simulink model "tqdtqr_rebuild_V3"  (R2021b)
settings: Solver=VariableStepAuto  StartTime=0.0  StopTime=10.0  RelTol=1e-3
undefined symbols (not defined in the file): ATQD_AfterTqMinGain_X_Deg, ATQD_APSCreepBaseTqD_X_kph, ATQD_APSCreepBaseTqD_Y_Deg, ATQD_APSCreepBaseTqR_X_kph, ATQD_APSCreepBaseTqR_Y_Deg, ATQD_APSCreepIterm_X_kph, ATQD_APSCreepIterm_Y_kph, ATQD_APSCreepPterm_X_kph, ATQD_APSCreepPterm_Y_kph, ATQD_APSDecReq_X_kph, ATQD_APSDecReq_Y_mps2, ATQD_APSDecReqCMD_X_kph, ATQD_APSDecReqTs_X_pct, ATQD_APSDecTimeGain_X_Deg, ATQD_APSDecTimeGain_Y_s, ATQD_APSReqLowSpd_X_Deg, ATQD_AutoHoldReleaseBPS_X_Deg, ATQD_AWDLoadTrqnsGain_X_kg, ATQD_AWDLoadTrqnsGain_Y_pct, ATQD_BOSEnBPSPosn_X_kph, ATQD_BOSMap_X_rpm, ATQD_BOSMap_Y_pct, ATQD_CreepBaseTqD_X_kph, ATQD_CreepBaseTqD_Y_Deg, ATQD_CreepBaseTqR_X_kph, ATQD_CreepBaseTqR_Y_Deg, ATQD_CreepBPSDisPosn_X_Deg, ATQD_CreepBPSDisPosnR_X_Deg, ATQD_CreepBPSEnPosn_X_Deg, ATQD_CreepBPSEnPosnR_X_Deg, ATQD_CreepDeltaTq_X_kph, ATQD_CreepIterm_X_kph, ATQD_CreepIterm_Y_kph, ATQD_CreepItermMaxLimit_X_pct, ATQD_CreepPreloadTime_X_kph, ATQD_CreepPreloadTq_X_kph, ATQD_CreepPreloadTq_Y_s, ATQD_CreepProtTq_X_Deg, ATQD_CreepPterm_X_kph, ATQD_CreepPterm_Y_kph, ATQD_CreepRrTqSpRat_X_rpm, ATQD_CreepRrTqSpRat_Y_Nm, ATQD_CreepTargetSpdD_X_pct, ATQD_CreepTargetSpdR_X_pct, ATQD_CreepUpLimitTq_X_rpm, ATQD_DecIneOPDHoldEnDelay_X_Deg, ATQD_DecIneOPDHoldEnDelay_Y_bar, ATQD_ECOTqMapD_X_rpm, ATQD_ECOTqMapD_Y_pct, ATQD_EMTqMapD_X_rpm, ATQD_EMTqMapD_Y_pct, ATQD_EOPDTqMapDCon_X_rpm, ATQD_EOPDTqMapDCon_Y_Deg, ATQD_EstInitVehWeight_X_c, ATQD_FAfterTqCMDGain_X_rpm, ATQD_FAfterTqCMDGain_Y_pct, ATQD_ForceLowSpd_X_Deg, ATQD_ForcePLimitSpd_X_Deg, ATQD_FrLossMAPLowV_X_rpm, ATQD_FrLossMAPLowV_Y_Nm ... (+949)
libraries: simulink x235, hcu_lib x208, tqr x63, tqd x6
(part 27 of 37)

== system tqdtqr_rebuild_V3/Input_Convert/Main function/Front//Rear ramp parameters determine/Front wheel rate limit determination/VTQR_VMCFEDUIncDec_Nm ==
  VTQR_FEDUWhlTqReqSmoothDelay_Nm : Inport
  VTQD_TqTargetShaftSpd_rpm : Inport  Port=2
  Action Port : ActionPort  ActionPortLabel=elseif(u4~=0)
  Data Type Conversion1 : DataTypeConversion  OutDataTypeStr=single
  Data Type Conversion2 : DataTypeConversion  OutDataTypeStr=single
  Data Type Conversion3 : DataTypeConversion  OutDataTypeStr=single
  MTQR_VMCFEDUTqDecSR_Z_Nm1 : Lookup_n-D  BreakpointsForDimension1=ATQR_VMCFEDUTqIncSR_Y_Nm  BreakpointsForDimension2=ATQR_VMCFEDUTqIncSR_X_rpm  Table=MTQR_VMCFEDUTqDecSR_Z_Nm  ExtrapMethod=Clip  InternalRulePriority=Speed  RndMeth=Simplest  InputSameDT=on
      settings: InputPortMap=u0,u1
  MTQR_VMCFEDUTqIncSR_Z_Nm1 : Lookup_n-D  BreakpointsForDimension1=ATQR_VMCFEDUTqIncSR_Y_Nm  BreakpointsForDimension2=ATQR_VMCFEDUTqIncSR_X_rpm  Table=MTQR_VMCFEDUTqIncSR_Z_Nm  ExtrapMethod=Clip  InternalRulePriority=Speed  RndMeth=Simplest  InputSameDT=on
      settings: InputPortMap=u0,u1
  Mux : Mux  Inputs=2
  VTQR_VMCFEDUIncDec_Nm : Outport
  VTQR_VMCFEDUIncDec_Nm1 : Outport  Port=2
  wires:
  [VTQD_TqTargetShaftSpd_rpm] -> MTQR_VMCFEDUTqDecSR_Z_Nm1/2
  [VTQR_FEDUWhlTqReqSmoothDelay_Nm] -> MTQR_VMCFEDUTqDecSR_Z_Nm1/1
  [VTQD_TqTargetShaftSpd_rpm] -> MTQR_VMCFEDUTqIncSR_Z_Nm1/2
  [VTQR_FEDUWhlTqReqSmoothDelay_Nm] -> MTQR_VMCFEDUTqIncSR_Z_Nm1/1
  VTQR_FEDUWhlTqReqSmoothDelay_Nm/1 -> [VTQR_FEDUWhlTqReqSmoothDelay_Nm]
  VTQD_TqTargetShaftSpd_rpm/1 -> [VTQD_TqTargetShaftSpd_rpm]
  [VTQR_VMCFEDUTqIncSR_Nm] -> Data Type Conversion1/1
  [VTQR_VMCFEDUTqDecSR_Nm] -> Data Type Conversion2/1
  Mux/1 -> VTQR_VMCFEDUIncDec_Nm/1
  MTQR_VMCFEDUTqIncSR_Z_Nm1/1 -> [VTQR_VMCFEDUTqIncSR_Nm]  "VTQR_VMCFEDUTqIncSR_Nm"
  MTQR_VMCFEDUTqDecSR_Z_Nm1/1 -> [VTQR_VMCFEDUTqDecSR_Nm]  "VTQR_VMCFEDUTqDecSR_Nm"
  Data Type Conversion2/1 -> Mux/2
  Data Type Conversion1/1 -> Mux/1
  Data Type Conversion3/1 -> VTQR_VMCFEDUIncDec_Nm1/1
  [VTQR_VMCFEDUTqDecSR_Nm] -> Data Type Conversion3/1

== system tqdtqr_rebuild_V3/Input_Convert/Main function/Front//Rear ramp parameters determine/Rear First order filter input tau map and determination/VTQR_CreepREDUTs_c ==
  VTQR_REDUWhlTqReqSmooth_Nm : Inport
  VTQD_TqTargetShaftSpd_rpm : Inport  Port=2
  VVMC_EstSlope_Deg : Inport  Port=3
  Action Port : ActionPort  ActionPortLabel=elseif(u2 ~= 0)
  Data Type Conversion : DataTypeConversion  OutDataTypeStr=single
  Data Type Conversion1 : DataTypeConversion  OutDataTypeStr=single
  MTQR_CreepGradeREDUTs_Z_c : Lookup_n-D  BreakpointsForDimension1=ATQR_CreepGradeREDUTs_Y_Deg  BreakpointsForDimension2=ATQR_CreepGradeREDUTs_X_rpm  Table=MTQR_CreepGradeREDUTs_Z_c  ExtrapMethod=Clip  InternalRulePriority=Speed  RndMeth=Simplest  InputSameDT=on
      settings: InputPortMap=u0,u1
  MTQR_CreepREDUTs_Z_c1 : Lookup_n-D  BreakpointsForDimension1=ATQR_CreepFEDUTs_Y_Nm  BreakpointsForDimension2=ATQR_CreepFEDUTs_X_rpm  Table=MTQR_CreepREDUTs_Z_c  ExtrapMethod=Clip  InternalRulePriority=Speed  RndMeth=Simplest  InputSameDT=on
      settings: InputPortMap=u0,u1
  Min : MinMax  Inputs=2
  VTQR_CreepREDUTs_c : Outport
  wires:
  [VTQR_CreepREDUTs_c] -> Data Type Conversion/1
  MTQR_CreepREDUTs_Z_c1/1 -> [VTQR_CreepREDUTs_c]  "VTQR_CreepREDUTs_c"
  VTQR_REDUWhlTqReqSmooth_Nm/1 -> [VTQR_REDUWhlTqReqSmooth_Nm]
  VTQD_TqTargetShaftSpd_rpm/1 -> [VTQD_TqTargetShaftSpd_rpm]
  VVMC_EstSlope_Deg/1 -> [VVMC_EstSlope_Deg]
  [VTQD_TqTargetShaftSpd_rpm] -> MTQR_CreepREDUTs_Z_c1/2
  [VTQR_REDUWhlTqReqSmooth_Nm] -> MTQR_CreepREDUTs_Z_c1/1
  [VTQD_TqTargetShaftSpd_rpm] -> MTQR_CreepGradeREDUTs_Z_c/2
  MTQR_CreepGradeREDUTs_Z_c/1 -> [VTQR_CreepGradeREDUTs_c]  "VTQR_CreepGradeREDUTs_c"
  [VVMC_EstSlope_Deg] -> MTQR_CreepGradeREDUTs_Z_c/1
  [VTQR_CreepGradeREDUTs_c] -> Data Type Conversion1/1
  Data Type Conversion/1 -> Min/1
  Data Type Conversion1/1 -> Min/2
  Min/1 -> VTQR_CreepREDUTs_c/1

== system tqdtqr_rebuild_V3/Input_Convert/Main function/Front//Rear ramp parameters determine/Rear First order filter input tau map and determination/VTQR_PreLoadPreEnTs_c ==
  KTQR_PreLoadPreEnTs_c : Inport
  Action Port : ActionPort  ActionPortLabel=elseif(u6~=0)
  VTQR_PreLoadPreEnTs_c : Outport
  wires:
  KTQR_PreLoadPreEnTs_c/1 -> VTQR_PreLoadPreEnTs_c/1

== system tqdtqr_rebuild_V3/Input_Convert/Main function/Front//Rear ramp parameters determine/Rear First order filter input tau map and determination/VTQR_PreLoadTs_c ==
  KTQR_PreLoadTs_c : Inport
  Action Port : ActionPort  ActionPortLabel=elseif(u5~=0)
  VTQR_PreLoadTs_c : Outport
  wires:
  KTQR_PreLoadTs_c/1 -> VTQR_PreLoadTs_c/1

== system tqdtqr_rebuild_V3/Input_Convert/Main function/Front//Rear ramp parameters determine/Rear First order filter input tau map and determination/VTQR_RDCActiveREDUTs_c ==
  VTQD_RegenMode_enum : Inport
  VVMC_ActMaxSlideRate_pct : Inport  Port=2
  Action Port : ActionPort  ActionPortLabel=if(u1~= 0)
  Data Type Conversion : DataTypeConversion  OutDataTypeStr=single
  Data Type Conversion1 : DataTypeConversion  OutDataTypeStr=single
  MTQR_AltRDCActiveREDUTs_Z_c1 : Lookup_n-D  BreakpointsForDimension1=ATQR_AltRDCActiveREDUTs_Y_enum  BreakpointsForDimension2=ATQR_AltRDCActiveREDUTs_X_pct  Table=MTQR_AltRDCActiveREDUTs_Z_c  TableDataTypeStr=Inherit: Inherit from 'Table data'  ExtrapMethod=Clip  InternalRulePriority=Speed  RndMeth=Simplest  InputSameDT=on
      settings: InputPortMap=u0,u1
  VTQR_RDCActiveREDUTs_c : Outport
  wires:
  MTQR_AltRDCActiveREDUTs_Z_c1/1 -> [VTQR_RDCActiveREDUTs_c]  "VTQR_RDCActiveREDUTs_c"
  Data Type Conversion1/1 -> MTQR_AltRDCActiveREDUTs_Z_c1/1
  VTQD_RegenMode_enum/1 -> Data Type Conversion1/1
  VVMC_ActMaxSlideRate_pct/1 -> MTQR_AltRDCActiveREDUTs_Z_c1/2
  [VTQR_RDCActiveREDUTs_c] -> Data Type Conversion/1
  Data Type Conversion/1 -> VTQR_RDCActiveREDUTs_c/1

== system tqdtqr_rebuild_V3/Input_Convert/Main function/Front//Rear ramp parameters determine/Rear First order filter input tau map and determination/VTQR_REDUTIPOutTs_c ==
  VTQD_TqTargetShaftSpd_rpm : Inport
  Action Port : ActionPort  ActionPortLabel=elseif(u4~=0)
  Data Type Conversion : DataTypeConversion  OutDataTypeStr=single
  MTQR_REDUTIPOutTs_Y_c1 : Lookup_n-D  NumberOfTableDimensions=1  BreakpointsForDimension1=ATQR_FEDUTIPOutTs_X_rpm  Table=MTQR_REDUTIPOutTs_Y_c  ExtrapMethod=Clip  InternalRulePriority=Speed  RndMeth=Simplest  InputSameDT=on
  VTQR_REDUTIPOutTs_c : Outport
  wires:
  MTQR_REDUTIPOutTs_Y_c1/1 -> [VTQR_REDUTIPOutTs_c]  "VTQR_REDUTIPOutTs_c"
  VTQD_TqTargetShaftSpd_rpm/1 -> MTQR_REDUTIPOutTs_Y_c1/1
  [VTQR_REDUTIPOutTs_c] -> Data Type Conversion/1
  Data Type Conversion/1 -> VTQR_REDUTIPOutTs_c/1

== system tqdtqr_rebuild_V3/Input_Convert/Main function/Front//Rear ramp parameters determine/Rear First order filter input tau map and determination/VTQR_REDUTs_c ==
  VTQR_REDUTs_c : Inport
  Action Port : ActionPort  ActionPortLabel=else
  VTQR_OutREDUTs_c : Outport
  wires:
  VTQR_REDUTs_c/1 -> VTQR_OutREDUTs_c/1

== system tqdtqr_rebuild_V3/Input_Convert/Main function/Front//Rear ramp parameters determine/Rear First order filter input tau map and determination/VTQR_VMCREDUTs_c ==
  VTQR_REDUWhlTqReqSmooth_Nm : Inport
  VTQD_TqTargetShaftSpd_rpm : Inport  Port=2
  Action Port : ActionPort  ActionPortLabel=elseif( u3 ~= 0)
  Data Type Conversion : DataTypeConversion  OutDataTypeStr=single
  MTQR_VMCREDUTs_Z_c1 : Lookup_n-D  BreakpointsForDimension1=ATQR_VMCREDUTs_Y_Nm  BreakpointsForDimension2=ATQR_VMCFEDUTs_X_rpm  Table=MTQR_VMCREDUTs_Z_c  ExtrapMethod=Clip  InternalRulePriority=Speed  RndMeth=Simplest  InputSameDT=on
      settings: InputPortMap=u0,u1
  VTQR_VMCREDUTs_c : Outport
  wires:
  [VTQR_VMCREDUTs_c] -> Data Type Conversion/1
  Data Type Conversion/1 -> VTQR_VMCREDUTs_c/1
  MTQR_VMCREDUTs_Z_c1/1 -> [VTQR_VMCREDUTs_c]  "VTQR_VMCREDUTs_c"
  VTQR_REDUWhlTqReqSmooth_Nm/1 -> MTQR_VMCREDUTs_Z_c1/1
  VTQD_TqTargetShaftSpd_rpm/1 -> MTQR_VMCREDUTs_Z_c1/2

== system tqdtqr_rebuild_V3/Input_Convert/Main function/Front//Rear ramp parameters determine/Rear wheel rate limit determination1/Drive mode ==
  VTQR_DriveModeTqIncDec_Nm : Inport
  Action Port : ActionPort  ActionPortLabel=else
  VTQR_OutDriveModeTqIncDec_Nm : Outport
  wires:
  VTQR_DriveModeTqIncDec_Nm/1 -> VTQR_OutDriveModeTqIncDec_Nm/1

== system tqdtqr_rebuild_V3/Input_Convert/Main function/Front//Rear ramp parameters determine/Rear wheel rate limit determination1/VTQD_OutRrZeroPointIncDec_Nm ==
  VTQD_RrZeroPointIncDec_Nm : Inport
  Action Port : ActionPort  ActionPortLabel=if(u1~= 0)
  VTQD_OutRrZeroPointIncDec_Nm : Outport
  wires:
  VTQD_RrZeroPointIncDec_Nm/1 -> VTQD_OutRrZeroPointIncDec_Nm/1

== system tqdtqr_rebuild_V3/Input_Convert/Main function/Front//Rear ramp parameters determine/Rear wheel rate limit determination1/VTQR_CreepREDUTqIncDecSR_Nm ==
  VTQR_REDUWhlTqReqSmoothDelay_Nm : Inport
  VTQD_TqTargetShaftSpd_rpm : Inport  Port=2
  VVMC_EstSlope_Deg : Inport  Port=3
  Action Port : ActionPort  ActionPortLabel=elseif(u2 ~= 0)
  Data Type Conversion : DataTypeConversion  OutDataTypeStr=single
  Data Type Conversion1 : DataTypeConversion  OutDataTypeStr=single
  MTQR_CreepGradeRTqDecSR_Z_c : Lookup_n-D  BreakpointsForDimension1=ATQR_CreepGradeRTqIncSR_Y_Deg  BreakpointsForDimension2=ATQR_CreepGradeRTqIncSR_X_rpm  Table=MTQR_CreepGradeRTqDecSR_Z_c  ExtrapMethod=Clip  InternalRulePriority=Speed  RndMeth=Simplest  InputSameDT=on
      settings: InputPortMap=u0,u1
  MTQR_CreepGradeRTqIncSR_Z_c : Lookup_n-D  BreakpointsForDimension1=ATQR_CreepGradeRTqIncSR_Y_Deg  BreakpointsForDimension2=ATQR_CreepGradeRTqIncSR_X_rpm  Table=MTQR_CreepGradeRTqIncSR_Z_c  ExtrapMethod=Clip  InternalRulePriority=Speed  RndMeth=Simplest  InputSameDT=on
      settings: InputPortMap=u0,u1
  MTQR_CreepREDUTqDecSR_Z_Nm1 : Lookup_n-D  BreakpointsForDimension1=ATQR_CreepFEDUTqIncSR_Y_Nm  BreakpointsForDimension2=ATQR_CreepFEDUTqIncSR_X_rpm  Table=MTQR_CreepREDUTqDecSR_Z_Nm  ExtrapMethod=Clip  InternalRulePriority=Speed  RndMeth=Simplest  InputSameDT=on
      settings: InputPortMap=u0,u1
  MTQR_CreepREDUTqIncSR_Z_Nm1 : Lookup_n-D  BreakpointsForDimension1=ATQR_CreepFEDUTqIncSR_Y_Nm  BreakpointsForDimension2=ATQR_CreepFEDUTqIncSR_X_rpm  Table=MTQR_CreepREDUTqIncSR_Z_Nm  ExtrapMethod=Clip  InternalRulePriority=Speed  RndMeth=Simplest  InputSameDT=on
      settings: InputPortMap=u0,u1
  Mux : Mux  Inputs=2
  Product : Product
  Product1 : Product
  VTQR_CreepREDUTqIncDecSR_Nm : Outport
  wires:
  VTQR_REDUWhlTqReqSmoothDelay_Nm/1 -> [VTQR_REDUWhlTqReqSmoothDelay_Nm]
  VTQD_TqTargetShaftSpd_rpm/1 -> [VTQD_TqTargetShaftSpd_rpm]
  [VTQD_TqTargetShaftSpd_rpm] -> MTQR_CreepREDUTqIncSR_Z_Nm1/2
  [VTQR_REDUWhlTqReqSmoothDelay_Nm] -> MTQR_CreepREDUTqIncSR_Z_Nm1/1
  [VTQR_REDUWhlTqReqSmoothDelay_Nm] -> MTQR_CreepREDUTqDecSR_Z_Nm1/1
  [VTQD_TqTargetShaftSpd_rpm] -> MTQR_CreepREDUTqDecSR_Z_Nm1/2
  [VTQR_CreepREDUTqIncSR_Nm] -> Data Type Conversion/1
  [VTQR_CreepREDUTqDecSR_Nm] -> Data Type Conversion1/1
  Data Type Conversion/1 -> Mux/1
  Data Type Conversion1/1 -> Mux/2
  Mux/1 -> VTQR_CreepREDUTqIncDecSR_Nm/1
  MTQR_CreepREDUTqIncSR_Z_Nm1/1 -> Product1/1
  [VTQR_CreepGradeRTqIncSR_c] -> Product1/2
  Product1/1 -> [VTQR_CreepREDUTqIncSR_Nm]  "VTQR_CreepREDUTqIncSR_Nm"
  [VVMC_EstSlope_Deg] -> MTQR_CreepGradeRTqDecSR_Z_c/1
  [VVMC_EstSlope_Deg] -> MTQR_CreepGradeRTqIncSR_Z_c/1
  [VTQD_TqTargetShaftSpd_rpm] -> MTQR_CreepGradeRTqDecSR_Z_c/2
  MTQR_CreepGradeRTqDecSR_Z_c/1 -> [VTQR_CreepGradeRTqDecSR_c]  "VTQR_CreepGradeRTqDecSR_c"
  MTQR_CreepGradeRTqIncSR_Z_c/1 -> [VTQR_CreepGradeRTqIncSR_c]  "VTQR_CreepGradeRTqIncSR_c"
  [VTQD_TqTargetShaftSpd_rpm] -> MTQR_CreepGradeRTqIncSR_Z_c/2
  Product/1 -> [VTQR_CreepREDUTqDecSR_Nm]  "VTQR_CreepREDUTqDecSR_Nm"
  MTQR_CreepREDUTqDecSR_Z_Nm1/1 -> Product/1
  [VTQR_CreepGradeRTqDecSR_c] -> Product/2
  VVMC_EstSlope_Deg/1 -> [VVMC_EstSlope_Deg]

== system tqdtqr_rebuild_V3/Input_Convert/Main function/Front//Rear ramp parameters determine/Rear wheel rate limit determination1/VTQR_RrPreLoadTqIncDecSR_Nm ==
  VTQR_REDUWhlTqReqSmoothDelay_Nm : Inport
  VTQD_TqTargetShaftSpd_rpm : Inport  Port=2
  Action Port : ActionPort  ActionPortLabel=elseif( u3 ~= 0)
  Data Type Conversion : DataTypeConversion  OutDataTypeStr=single
  Data Type Conversion1 : DataTypeConversion  OutDataTypeStr=single
  MTQR_RrPreLoadTqDecSR_Z_Nm1 : Lookup_n-D  BreakpointsForDimension1=ATQR_RrPreLoadTqIncSR_Y_Nm  BreakpointsForDimension2=ATQR_RrPreLoadTqIncSR_X_rpm  Table=MTQR_RrPreLoadTqDecSR_Z_Nm  ExtrapMethod=Clip  InternalRulePriority=Speed  RndMeth=Simplest  InputSameDT=on
      settings: InputPortMap=u0,u1
  MTQR_RrPreLoadTqIncSR_Z_Nm1 : Lookup_n-D  BreakpointsForDimension1=ATQR_RrPreLoadTqIncSR_Y_Nm  BreakpointsForDimension2=ATQR_RrPreLoadTqIncSR_X_rpm  Table=MTQR_RrPreLoadTqIncSR_Z_Nm  ExtrapMethod=Clip  InternalRulePriority=Speed  RndMeth=Simplest  InputSameDT=on
      settings: InputPortMap=u0,u1
  Mux : Mux  Inputs=2
  VTQR_RrPreLoadTqIncDecSR_Nm : Outport
  wires:
  Mux/1 -> VTQR_RrPreLoadTqIncDecSR_Nm/1
  Data Type Conversion1/1 -> Mux/2
  Data Type Conversion/1 -> Mux/1
  [VTQR_RrPreLoadTqDecSR_Nm] -> Data Type Conversion1/1
  [VTQR_RrPreLoadTqIncSR_Nm] -> Data Type Conversion/1
  VTQD_TqTargetShaftSpd_rpm/1 -> [VTQD_TqTargetShaftSpd_rpm]
  VTQR_REDUWhlTqReqSmoothDelay_Nm/1 -> [VTQR_REDUWhlTqReqSmoothDelay_Nm]
  MTQR_RrPreLoadTqIncSR_Z_Nm1/1 -> [VTQR_RrPreLoadTqIncSR_Nm]  "VTQR_RrPreLoadTqIncSR_Nm"
  MTQR_RrPreLoadTqDecSR_Z_Nm1/1 -> [VTQR_RrPreLoadTqDecSR_Nm]  "VTQR_RrPreLoadTqDecSR_Nm"
  [VTQR_REDUWhlTqReqSmoothDelay_Nm] -> MTQR_RrPreLoadTqIncSR_Z_Nm1/1
  [VTQD_TqTargetShaftSpd_rpm] -> MTQR_RrPreLoadTqIncSR_Z_Nm1/2
  [VTQR_REDUWhlTqReqSmoothDelay_Nm] -> MTQR_RrPreLoadTqDecSR_Z_Nm1/1
  [VTQD_TqTargetShaftSpd_rpm] -> MTQR_RrPreLoadTqDecSR_Z_Nm1/2

== system tqdtqr_rebuild_V3/Input_Convert/Main function/Front//Rear ramp parameters determine/Rear wheel rate limit determination1/VTQR_VMCREDUTqIncDecSR_Nm ==
  VTQR_REDUWhlTqReqSmoothDelay_Nm : Inport
  VTQD_TqTargetShaftSpd_rpm : Inport  Port=2
  Action Port : ActionPort  ActionPortLabel=elseif( u4~=0)
  Data Type Conversion : DataTypeConversion  OutDataTypeStr=single
  Data Type Conversion1 : DataTypeConversion  OutDataTypeStr=single
  MTQR_VMCREDUTqDecSR_Z_Nm1 : Lookup_n-D  BreakpointsForDimension1=ATQR_VMCREDUTqIncSR_Y_Nm  BreakpointsForDimension2=ATQR_VMCFEDUTqIncSR_X_rpm  Table=MTQR_VMCREDUTqDecSR_Z_Nm  ExtrapMethod=Clip  InternalRulePriority=Speed  RndMeth=Simplest  InputSameDT=on
      settings: InputPortMap=u0,u1
  MTQR_VMCREDUTqIncSR_Z_Nm1 : Lookup_n-D  BreakpointsForDimension1=ATQR_VMCREDUTqIncSR_Y_Nm  BreakpointsForDimension2=ATQR_VMCFEDUTqIncSR_X_rpm  Table=MTQR_VMCREDUTqIncSR_Z_Nm  ExtrapMethod=Clip  InternalRulePriority=Speed  RndMeth=Simplest  InputSameDT=on
      settings: InputPortMap=u0,u1
  Mux : Mux  Inputs=2
  VTQR_VMCREDUTqIncDecSR_Nm : Outport
  VTQR_VMCREDUTqDecSR_Nm : Outport  Port=2
  wires:
  [VTQD_TqTargetShaftSpd_rpm] -> MTQR_VMCREDUTqDecSR_Z_Nm1/2
  [VTQR_REDUWhlTqReqSmoothDelay_Nm] -> MTQR_VMCREDUTqDecSR_Z_Nm1/1
  [VTQD_TqTargetShaftSpd_rpm] -> MTQR_VMCREDUTqIncSR_Z_Nm1/2
  [VTQR_REDUWhlTqReqSmoothDelay_Nm] -> MTQR_VMCREDUTqIncSR_Z_Nm1/1
  VTQR_REDUWhlTqReqSmoothDelay_Nm/1 -> [VTQR_REDUWhlTqReqSmoothDelay_Nm]
  VTQD_TqTargetShaftSpd_rpm/1 -> [VTQD_TqTargetShaftSpd_rpm]
  [VTQR_VMCREDUTqIncSR_Nm] -> Data Type Conversion/1
  [VTQR_VMCREDUTqDecSR_Nm] -> Data Type Conversion1/1
  Data Type Conversion/1 -> Mux/1
  Data Type Conversion1/1 -> Mux/2
  Mux/1 -> VTQR_VMCREDUTqIncDecSR_Nm/1
  MTQR_VMCREDUTqDecSR_Z_Nm1/1 -> [VTQR_VMCREDUTqDecSR_Nm]  "VTQR_VMCREDUTqDecSR_Nm"
  MTQR_VMCREDUTqIncSR_Z_Nm1/1 -> [VTQR_VMCREDUTqIncSR_Nm]  "VTQR_VMCREDUTqIncSR_Nm"
  [VTQR_VMCREDUTqDecSR_Nm] -> VTQR_VMCREDUTqDecSR_Nm/1

== system tqdtqr_rebuild_V3/Input_Convert/Main function/Front//Rear zero point transfer/Negative Rate limit Determination/VTQR_FrNegRateLimitDecE_Nm ==
  VTQD_TqTargetShaftSpd_rpm : Inport
  VTQR_FEDUWhlTqReqSmoothDelay_Nm : Inport  Port=2
  Action Port : ActionPort  ActionPortLabel=elseif(u2 ~= 0)
  MTQR_FrNegRateLimitDecE_Z_Nm : Lookup_n-D  BreakpointsForDimension1=ATQR_FrNegRateLimitIncN_Y_Nm  BreakpointsForDimension2=ATQR_FrNegRateLimitIncN_X_rpm  Table=MTQR_FrNegRateLimitDecE_Z_Nm  ExtrapMethod=Clip  UseLastTableValue=on  InternalRulePriority=Speed  RndMeth=Simplest  InputSameDT=on
      settings: InputPortMap=u0,u1
  VTQR_FrNegRateLimitDecE_Nm : Outport
  wires:
  VTQD_TqTargetShaftSpd_rpm/1 -> MTQR_FrNegRateLimitDecE_Z_Nm/2
  VTQR_FEDUWhlTqReqSmoothDelay_Nm/1 -> MTQR_FrNegRateLimitDecE_Z_Nm/1
  MTQR_FrNegRateLimitDecE_Z_Nm/1 -> VTQR_FrNegRateLimitDecE_Nm/1  "VTQR_FrNegRateLimitDecE_Nm"

== system tqdtqr_rebuild_V3/Input_Convert/Main function/Front//Rear zero point transfer/Negative Rate limit Determination/VTQR_FrNegRateLimitDecN_Nm ==
  VTQD_TqTargetShaftSpd_rpm : Inport
  VTQR_FEDUWhlTqReqSmoothDelay_Nm : Inport  Port=2
  Action Port : ActionPort  ActionPortLabel=if(u1~= 0)
  MTQR_FrNegRateLimitDecN_Z_Nm : Lookup_n-D  BreakpointsForDimension1=ATQR_FrNegRateLimitIncN_Y_Nm  BreakpointsForDimension2=ATQR_FrNegRateLimitIncN_X_rpm  Table=MTQR_FrNegRateLimitDecN_Z_Nm  ExtrapMethod=Clip  UseLastTableValue=on  InternalRulePriority=Speed  RndMeth=Simplest  InputSameDT=on
      settings: InputPortMap=u0,u1
  VTQR_FrNegRateLimitDecN_Nm : Outport
  wires:
  VTQD_TqTargetShaftSpd_rpm/1 -> MTQR_FrNegRateLimitDecN_Z_Nm/2
  VTQR_FEDUWhlTqReqSmoothDelay_Nm/1 -> MTQR_FrNegRateLimitDecN_Z_Nm/1
  MTQR_FrNegRateLimitDecN_Z_Nm/1 -> VTQR_FrNegRateLimitDecN_Nm/1  "VTQR_FrNegRateLimitDecN_Nm"

== system tqdtqr_rebuild_V3/Input_Convert/Main function/Front//Rear zero point transfer/Negative Rate limit Determination/VTQR_FrNegRateLimitDecS_Nm ==
  VTQD_TqTargetShaftSpd_rpm : Inport
  VTQR_FEDUWhlTqReqSmoothDelay_Nm : Inport  Port=2
  Action Port : ActionPort  ActionPortLabel=elseif( u3 ~= 0)
  MTQR_FrNegRateLimitDecS_Z_Nm : Lookup_n-D  BreakpointsForDimension1=ATQR_FrNegRateLimitIncN_Y_Nm  BreakpointsForDimension2=ATQR_FrNegRateLimitIncN_X_rpm  Table=MTQR_FrNegRateLimitDecS_Z_Nm  ExtrapMethod=Clip  UseLastTableValue=on  InternalRulePriority=Speed  RndMeth=Simplest  InputSameDT=on
      settings: InputPortMap=u0,u1
  VTQR_FrNegRateLimitDecS_Nm : Outport
  wires:
  VTQR_FEDUWhlTqReqSmoothDelay_Nm/1 -> MTQR_FrNegRateLimitDecS_Z_Nm/1
  VTQD_TqTargetShaftSpd_rpm/1 -> MTQR_FrNegRateLimitDecS_Z_Nm/2
  MTQR_FrNegRateLimitDecS_Z_Nm/1 -> VTQR_FrNegRateLimitDecS_Nm/1  "VTQR_FrNegRateLimitDecS_Nm"

== system tqdtqr_rebuild_V3/Input_Convert/Main function/Front//Rear zero point transfer/Negative Rate limit Determination/VTQR_FrNegRateLimitIncE_Nm ==
  VTQD_TqTargetShaftSpd_rpm : Inport
  VTQR_FEDUWhlTqReqSmoothDelay_Nm : Inport  Port=2
  Action Port : ActionPort  ActionPortLabel=elseif(u2 ~= 0)
  MTQR_FrNegRateLimitIncE_Z_Nm : Lookup_n-D  BreakpointsForDimension1=ATQR_FrNegRateLimitIncN_Y_Nm  BreakpointsForDimension2=ATQR_FrNegRateLimitIncN_X_rpm  Table=MTQR_FrNegRateLimitIncE_Z_Nm  ExtrapMethod=Clip  UseLastTableValue=on  InternalRulePriority=Speed  RndMeth=Simplest  InputSameDT=on
      settings: InputPortMap=u0,u1
  VTQR_FrNegRateLimitIncE_Nm : Outport
  wires:
  VTQD_TqTargetShaftSpd_rpm/1 -> MTQR_FrNegRateLimitIncE_Z_Nm/2
  VTQR_FEDUWhlTqReqSmoothDelay_Nm/1 -> MTQR_FrNegRateLimitIncE_Z_Nm/1
  MTQR_FrNegRateLimitIncE_Z_Nm/1 -> VTQR_FrNegRateLimitIncE_Nm/1  "VTQR_FrNegRateLimitIncE_Nm"

== system tqdtqr_rebuild_V3/Input_Convert/Main function/Front//Rear zero point transfer/Negative Rate limit Determination/VTQR_FrNegRateLimitIncN_Nm ==
  VTQD_TqTargetShaftSpd_rpm : Inport
  VTQR_FEDUWhlTqReqSmoothDelay_Nm : Inport  Port=2
  Action Port : ActionPort  ActionPortLabel=if(u1~= 0)
  MTQR_FrNegRateLimitIncN_Z_Nm : Lookup_n-D  BreakpointsForDimension1=ATQR_FrNegRateLimitIncN_Y_Nm  BreakpointsForDimension2=ATQR_FrNegRateLimitIncN_X_rpm  Table=MTQR_FrNegRateLimitIncN_Z_Nm  ExtrapMethod=Clip  UseLastTableValue=on  InternalRulePriority=Speed  RndMeth=Simplest  InputSameDT=on
      settings: InputPortMap=u0,u1
  VTQR_FrNegRateLimitIncN_Nm : Outport
  wires:
  VTQD_TqTargetShaftSpd_rpm/1 -> MTQR_FrNegRateLimitIncN_Z_Nm/2
  VTQR_FEDUWhlTqReqSmoothDelay_Nm/1 -> MTQR_FrNegRateLimitIncN_Z_Nm/1
  MTQR_FrNegRateLimitIncN_Z_Nm/1 -> VTQR_FrNegRateLimitIncN_Nm/1  "VTQR_FrNegRateLimitIncN_Nm"

== system tqdtqr_rebuild_V3/Input_Convert/Main function/Front//Rear zero point transfer/Negative Rate limit Determination/VTQR_FrNegRateLimitIncS_Nm ==
  VTQD_TqTargetShaftSpd_rpm : Inport
  VTQR_FEDUWhlTqReqSmoothDelay_Nm : Inport  Port=2
  Action Port : ActionPort  ActionPortLabel=elseif( u3 ~= 0)
  MTQR_FrNegRateLimitIncS_Z_Nm : Lookup_n-D  BreakpointsForDimension1=ATQR_FrNegRateLimitIncN_Y_Nm  BreakpointsForDimension2=ATQR_FrNegRateLimitIncN_X_rpm  Table=MTQR_FrNegRateLimitIncS_Z_Nm  ExtrapMethod=Clip  UseLastTableValue=on  InternalRulePriority=Speed  RndMeth=Simplest  InputSameDT=on
      settings: InputPortMap=u0,u1
  VTQR_FrNegRateLimitIncS_Nm : Outport
  wires:
  VTQR_FEDUWhlTqReqSmoothDelay_Nm/1 -> MTQR_FrNegRateLimitIncS_Z_Nm/1
  VTQD_TqTargetShaftSpd_rpm/1 -> MTQR_FrNegRateLimitIncS_Z_Nm/2
  MTQR_FrNegRateLimitIncS_Z_Nm/1 -> VTQR_FrNegRateLimitIncS_Nm/1  "VTQR_FrNegRateLimitIncS_Nm"

== system tqdtqr_rebuild_V3/Input_Convert/Main function/Front//Rear zero point transfer/Negative Rate limit Determination1/VTQR_RrNegRateLimitDecE_Nm ==
  VTQD_TqTargetShaftSpd_rpm : Inport
  VTQR_REDUWhlTqReqSmoothDelay_Nm : Inport  Port=2
  Action Port : ActionPort  ActionPortLabel=elseif(u2 ~= 0)
  MTQR_RrNegRateLimitDecE_Z_Nm : Lookup_n-D  BreakpointsForDimension1=ATQR_RrNegRateLimitIncN_Y_Nm  BreakpointsForDimension2=ATQR_RrNegRateLimitIncN_X_rpm  Table=MTQR_RrNegRateLimitDecE_Z_Nm  ExtrapMethod=Clip  UseLastTableValue=on  InternalRulePriority=Speed  RndMeth=Simplest  InputSameDT=on
      settings: InputPortMap=u0,u1
  VTQR_RrNegRateLimitDecE_Nm : Outport
  wires:
  MTQR_RrNegRateLimitDecE_Z_Nm/1 -> VTQR_RrNegRateLimitDecE_Nm/1  "VTQR_RrNegRateLimitDecE_Nm"
  VTQR_REDUWhlTqReqSmoothDelay_Nm/1 -> MTQR_RrNegRateLimitDecE_Z_Nm/1
  VTQD_TqTargetShaftSpd_rpm/1 -> MTQR_RrNegRateLimitDecE_Z_Nm/2

== system tqdtqr_rebuild_V3/Input_Convert/Main function/Front//Rear zero point transfer/Negative Rate limit Determination1/VTQR_RrNegRateLimitDecN_Nm ==
  VTQD_TqTargetShaftSpd_rpm : Inport
  VTQR_REDUWhlTqReqSmoothDelay_Nm : Inport  Port=2
  Action Port : ActionPort  ActionPortLabel=if(u1~= 0)
  MTQR_RrNegRateLimitDecN_Z_Nm : Lookup_n-D  BreakpointsForDimension1=ATQR_RrNegRateLimitIncN_Y_Nm  BreakpointsForDimension2=ATQR_RrNegRateLimitIncN_X_rpm  Table=MTQR_RrNegRateLimitDecN_Z_Nm  ExtrapMethod=Clip  UseLastTableValue=on  InternalRulePriority=Speed  RndMeth=Simplest  InputSameDT=on
      settings: InputPortMap=u0,u1
  VTQR_RrNegRateLimitDecN_Nm : Outport
  wires:
  MTQR_RrNegRateLimitDecN_Z_Nm/1 -> VTQR_RrNegRateLimitDecN_Nm/1  "VTQR_RrNegRateLimitDecN_Nm"
  VTQR_REDUWhlTqReqSmoothDelay_Nm/1 -> MTQR_RrNegRateLimitDecN_Z_Nm/1
  VTQD_TqTargetShaftSpd_rpm/1 -> MTQR_RrNegRateLimitDecN_Z_Nm/2

== system tqdtqr_rebuild_V3/Input_Convert/Main function/Front//Rear zero point transfer/Negative Rate limit Determination1/VTQR_RrNegRateLimitDecS_Nm ==
  VTQD_TqTargetShaftSpd_rpm : Inport
  VTQR_REDUWhlTqReqSmoothDelay_Nm : Inport  Port=2
  Action Port : ActionPort  ActionPortLabel=elseif( u3 ~= 0)
  MTQR_RrNegRateLimitDecE_Z_Nm : Lookup_n-D  BreakpointsForDimension1=ATQR_RrNegRateLimitIncN_Y_Nm  BreakpointsForDimension2=ATQR_RrNegRateLimitIncN_X_rpm  Table=MTQR_RrNegRateLimitDecS_Z_Nm  ExtrapMethod=Clip  UseLastTableValue=on  InternalRulePriority=Speed  RndMeth=Simplest  InputSameDT=on
      settings: InputPortMap=u0,u1
  VTQR_RrNegRateLimitDecS_Nm : Outport
  wires:
  MTQR_RrNegRateLimitDecE_Z_Nm/1 -> VTQR_RrNegRateLimitDecS_Nm/1  "VTQR_RrNegRateLimitDecS_Nm"
  VTQD_TqTargetShaftSpd_rpm/1 -> MTQR_RrNegRateLimitDecE_Z_Nm/2
  VTQR_REDUWhlTqReqSmoothDelay_Nm/1 -> MTQR_RrNegRateLimitDecE_Z_Nm/1

== system tqdtqr_rebuild_V3/Input_Convert/Main function/Front//Rear zero point transfer/Negative Rate limit Determination1/VTQR_RrNegRateLimitIncE_Nm ==
  VTQD_TqTargetShaftSpd_rpm : Inport
  VTQR_REDUWhlTqReqSmoothDelay_Nm : Inport  Port=2
  Action Port : ActionPort  ActionPortLabel=elseif(u2 ~= 0)
  MTQR_RrNegRateLimitIncE_Z_Nm : Lookup_n-D  BreakpointsForDimension1=ATQR_RrNegRateLimitIncN_Y_Nm  BreakpointsForDimension2=ATQR_RrNegRateLimitIncN_X_rpm  Table=MTQR_RrNegRateLimitIncE_Z_Nm  ExtrapMethod=Clip  UseLastTableValue=on  InternalRulePriority=Speed  RndMeth=Simplest  InputSameDT=on
      settings: InputPortMap=u0,u1
  VTQR_RrNegRateLimitIncE_Nm : Outport
  wires:
  MTQR_RrNegRateLimitIncE_Z_Nm/1 -> VTQR_RrNegRateLimitIncE_Nm/1  "VTQR_RrNegRateLimitIncE_Nm"
  VTQR_REDUWhlTqReqSmoothDelay_Nm/1 -> MTQR_RrNegRateLimitIncE_Z_Nm/1
  VTQD_TqTargetShaftSpd_rpm/1 -> MTQR_RrNegRateLimitIncE_Z_Nm/2

== system tqdtqr_rebuild_V3/Input_Convert/Main function/Front//Rear zero point transfer/Negative Rate limit Determination1/VTQR_RrNegRateLimitIncN_Nm ==
  VTQD_TqTargetShaftSpd_rpm : Inport
  VTQR_REDUWhlTqReqSmoothDelay_Nm : Inport  Port=2
  Action Port : ActionPort  ActionPortLabel=if(u1~= 0)
  MTQR_RrNegRateLimitIncN_Z_Nm : Lookup_n-D  BreakpointsForDimension1=ATQR_RrNegRateLimitIncN_Y_Nm  BreakpointsForDimension2=ATQR_RrNegRateLimitIncN_X_rpm  Table=MTQR_RrNegRateLimitIncN_Z_Nm  ExtrapMethod=Clip  UseLastTableValue=on  InternalRulePriority=Speed  RndMeth=Simplest  InputSameDT=on
      settings: InputPortMap=u0,u1
  VTQR_RrNegRateLimitIncN_Nm : Outport
  wires:
  MTQR_RrNegRateLimitIncN_Z_Nm/1 -> VTQR_RrNegRateLimitIncN_Nm/1  "VTQR_RrNegRateLimitIncN_Nm"
  VTQR_REDUWhlTqReqSmoothDelay_Nm/1 -> MTQR_RrNegRateLimitIncN_Z_Nm/1
  VTQD_TqTargetShaftSpd_rpm/1 -> MTQR_RrNegRateLimitIncN_Z_Nm/2

== system tqdtqr_rebuild_V3/Input_Convert/Main function/Front//Rear zero point transfer/Negative Rate limit Determination1/VTQR_RrNegRateLimitIncS_Nm ==
  VTQD_TqTargetShaftSpd_rpm : Inport
  VTQR_REDUWhlTqReqSmoothDelay_Nm : Inport  Port=2
  Action Port : ActionPort  ActionPortLabel=elseif( u3 ~= 0)
  MTQR_RrNegRateLimitIncS_Z_Nm : Lookup_n-D  BreakpointsForDimension1=ATQR_RrNegRateLimitIncN_Y_Nm  BreakpointsForDimension2=ATQR_RrNegRateLimitIncN_X_rpm  Table=MTQR_RrNegRateLimitIncS_Z_Nm  ExtrapMethod=Clip  UseLastTableValue=on  InternalRulePriority=Speed  RndMeth=Simplest  InputSameDT=on
      settings: InputPortMap=u0,u1
  VTQR_RrNegRateLimitIncS_Nm : Outport
  wires:
  MTQR_RrNegRateLimitIncS_Z_Nm/1 -> VTQR_RrNegRateLimitIncS_Nm/1  "VTQR_RrNegRateLimitIncS_Nm"
  VTQD_TqTargetShaftSpd_rpm/1 -> MTQR_RrNegRateLimitIncS_Z_Nm/2
  VTQR_REDUWhlTqReqSmoothDelay_Nm/1 -> MTQR_RrNegRateLimitIncS_Z_Nm/1

== system tqdtqr_rebuild_V3/Input_Convert/Main function/Front//Rear zero point transfer/Positive Rate limit Determination/VTQR_FrPosRateLimitDecE_Nm ==
  VTQD_TqTargetShaftSpd_rpm : Inport
  VTQR_FEDUWhlTqReqSmoothDelay_Nm : Inport  Port=2
  Action Port : ActionPort  ActionPortLabel=elseif(u2 ~= 0)
  MTQR_FrPosRateLimitDecE_Z_Nm : Lookup_n-D  BreakpointsForDimension1=ATQR_FrPosRateLimitIncN_Y_Nm  BreakpointsForDimension2=ATQR_FrPosRateLimitIncN_X_rpm  Table=MTQR_FrPosRateLimitDecE_Z_Nm  ExtrapMethod=Clip  UseLastTableValue=on  InternalRulePriority=Speed  RndMeth=Simplest  InputSameDT=on
      settings: InputPortMap=u0,u1
  VTQR_FrPosRateLimitDecE_Nm : Outport
  wires:
  MTQR_FrPosRateLimitDecE_Z_Nm/1 -> VTQR_FrPosRateLimitDecE_Nm/1  "VTQR_FrPosRateLimitDecE_Nm"
  VTQR_FEDUWhlTqReqSmoothDelay_Nm/1 -> MTQR_FrPosRateLimitDecE_Z_Nm/1
  VTQD_TqTargetShaftSpd_rpm/1 -> MTQR_FrPosRateLimitDecE_Z_Nm/2

== system tqdtqr_rebuild_V3/Input_Convert/Main function/Front//Rear zero point transfer/Positive Rate limit Determination/VTQR_FrPosRateLimitDecN_Nm ==
  VTQD_TqTargetShaftSpd_rpm : Inport
  VTQR_FEDUWhlTqReqSmoothDelay_Nm : Inport  Port=2
  Action Port : ActionPort  ActionPortLabel=if(u1~= 0)
  MTQR_FrPosRateLimitDecN_Z_Nm : Lookup_n-D  BreakpointsForDimension1=ATQR_FrPosRateLimitIncN_Y_Nm  BreakpointsForDimension2=ATQR_FrPosRateLimitIncN_X_rpm  Table=MTQR_FrPosRateLimitDecN_Z_Nm  ExtrapMethod=Clip  UseLastTableValue=on  InternalRulePriority=Speed  RndMeth=Simplest  InputSameDT=on
      settings: InputPortMap=u0,u1
  VTQR_FrPosRateLimitDecN_Nm : Outport
  wires:
  MTQR_FrPosRateLimitDecN_Z_Nm/1 -> VTQR_FrPosRateLimitDecN_Nm/1  "VTQR_FrPosRateLimitDecN_Nm"
  VTQR_FEDUWhlTqReqSmoothDelay_Nm/1 -> MTQR_FrPosRateLimitDecN_Z_Nm/1
  VTQD_TqTargetShaftSpd_rpm/1 -> MTQR_FrPosRateLimitDecN_Z_Nm/2

== system tqdtqr_rebuild_V3/Input_Convert/Main function/Front//Rear zero point transfer/Positive Rate limit Determination/VTQR_FrPosRateLimitDecS_Nm ==
  VTQD_TqTargetShaftSpd_rpm : Inport
  VTQR_FEDUWhlTqReqSmoothDelay_Nm : Inport  Port=2
  Action Port : ActionPort  ActionPortLabel=elseif( u3 ~= 0)
  MTQR_FrPosRateLimitDecS_Z_Nm : Lookup_n-D  BreakpointsForDimension1=ATQR_FrPosRateLimitIncN_Y_Nm  BreakpointsForDimension2=ATQR_FrPosRateLimitIncN_X_rpm  Table=MTQR_FrPosRateLimitDecS_Z_Nm  ExtrapMethod=Clip  UseLastTableValue=on  InternalRulePriority=Speed  RndMeth=Simplest  InputSameDT=on
      settings: InputPortMap=u0,u1
  VTQR_FrPosRateLimitDecS_Nm : Outport
  wires:
  MTQR_FrPosRateLimitDecS_Z_Nm/1 -> VTQR_FrPosRateLimitDecS_Nm/1  "VTQR_FrPosRateLimitDecS_Nm"
  VTQD_TqTargetShaftSpd_rpm/1 -> MTQR_FrPosRateLimitDecS_Z_Nm/2
  VTQR_FEDUWhlTqReqSmoothDelay_Nm/1 -> MTQR_FrPosRateLimitDecS_Z_Nm/1

== system tqdtqr_rebuild_V3/Input_Convert/Main function/Front//Rear zero point transfer/Positive Rate limit Determination/VTQR_FrPosRateLimitIncE_Nm ==
  VTQD_TqTargetShaftSpd_rpm : Inport
  VTQR_FEDUWhlTqReqSmoothDelay_Nm : Inport  Port=2
  Action Port : ActionPort  ActionPortLabel=elseif(u2 ~= 0)
  MTQR_FrPosRateLimitIncE_Z_Nm : Lookup_n-D  BreakpointsForDimension1=ATQR_FrPosRateLimitIncN_Y_Nm  BreakpointsForDimension2=ATQR_FrPosRateLimitIncN_X_rpm  Table=MTQR_FrPosRateLimitIncE_Z_Nm  ExtrapMethod=Clip  UseLastTableValue=on  InternalRulePriority=Speed  RndMeth=Simplest  InputSameDT=on
      settings: InputPortMap=u0,u1
  VTQR_FrPosRateLimitIncE_Nm : Outport
  wires:
  MTQR_FrPosRateLimitIncE_Z_Nm/1 -> VTQR_FrPosRateLimitIncE_Nm/1  "VTQR_FrPosRateLimitIncE_Nm"
  VTQR_FEDUWhlTqReqSmoothDelay_Nm/1 -> MTQR_FrPosRateLimitIncE_Z_Nm/1
  VTQD_TqTargetShaftSpd_rpm/1 -> MTQR_FrPosRateLimitIncE_Z_Nm/2

== system tqdtqr_rebuild_V3/Input_Convert/Main function/Front//Rear zero point transfer/Positive Rate limit Determination/VTQR_FrPosRateLimitIncN_Nm ==
  VTQD_TqTargetShaftSpd_rpm : Inport
  VTQR_FEDUWhlTqReqSmoothDelay_Nm : Inport  Port=2
  Action Port : ActionPort  ActionPortLabel=if(u1~= 0)
  MTQR_FrPosRateLimitIncN_Z_Nm : Lookup_n-D  BreakpointsForDimension1=ATQR_FrPosRateLimitIncN_Y_Nm  BreakpointsForDimension2=ATQR_FrPosRateLimitIncN_X_rpm  Table=MTQR_FrPosRateLimitIncN_Z_Nm  ExtrapMethod=Clip  UseLastTableValue=on  InternalRulePriority=Speed  RndMeth=Simplest  InputSameDT=on
      settings: InputPortMap=u0,u1
  VTQR_FrPosRateLimitIncN_Nm : Outport
  wires:
  MTQR_FrPosRateLimitIncN_Z_Nm/1 -> VTQR_FrPosRateLimitIncN_Nm/1  "VTQR_FrPosRateLimitIncN_Nm"
  VTQR_FEDUWhlTqReqSmoothDelay_Nm/1 -> MTQR_FrPosRateLimitIncN_Z_Nm/1
  VTQD_TqTargetShaftSpd_rpm/1 -> MTQR_FrPosRateLimitIncN_Z_Nm/2

== system tqdtqr_rebuild_V3/Input_Convert/Main function/Front//Rear zero point transfer/Positive Rate limit Determination/VTQR_FrPosRateLimitIncS_Nm ==
  VTQD_TqTargetShaftSpd_rpm : Inport
  VTQR_FEDUWhlTqReqSmoothDelay_Nm : Inport  Port=2
  Action Port : ActionPort  ActionPortLabel=elseif( u3 ~= 0)
  MTQR_FrPosRateLimitIncS_Z_Nm : Lookup_n-D  BreakpointsForDimension1=ATQR_FrPosRateLimitIncN_Y_Nm  BreakpointsForDimension2=ATQR_FrPosRateLimitIncN_X_rpm  Table=MTQR_FrPosRateLimitIncS_Z_Nm  ExtrapMethod=Clip  UseLastTableValue=on  InternalRulePriority=Speed  RndMeth=Simplest  InputSameDT=on
      settings: InputPortMap=u0,u1
  VTQR_FrPosRateLimitIncS_Nm : Outport
  wires:
  MTQR_FrPosRateLimitIncS_Z_Nm/1 -> VTQR_FrPosRateLimitIncS_Nm/1  "VTQR_FrPosRateLimitIncS_Nm"
  VTQD_TqTargetShaftSpd_rpm/1 -> MTQR_FrPosRateLimitIncS_Z_Nm/2
  VTQR_FEDUWhlTqReqSmoothDelay_Nm/1 -> MTQR_FrPosRateLimitIncS_Z_Nm/1

== system tqdtqr_rebuild_V3/Input_Convert/Main function/Front//Rear zero point transfer/Positive Rate limit Determination1/VTQR_RrPosRateLimitDecE_Nm ==
  VTQD_TqTargetShaftSpd_rpm : Inport
  VTQR_REDUWhlTqReqSmoothDelay_Nm : Inport  Port=2
  Action Port : ActionPort  ActionPortLabel=elseif(u2 ~= 0)
  MTQR_RrPosRateLimitDecE_Z_Nm : Lookup_n-D  BreakpointsForDimension1=ATQR_RrPosRateLimitIncN_Y_Nm  BreakpointsForDimension2=ATQR_RrPosRateLimitIncN_X_rpm  Table=MTQR_RrPosRateLimitDecE_Z_Nm  ExtrapMethod=Clip  UseLastTableValue=on  InternalRulePriority=Speed  RndMeth=Simplest  InputSameDT=on
      settings: InputPortMap=u0,u1
  VTQR_RrPosRateLimitDecE_Nm : Outport
  wires:
  VTQD_TqTargetShaftSpd_rpm/1 -> MTQR_RrPosRateLimitDecE_Z_Nm/2
  VTQR_REDUWhlTqReqSmoothDelay_Nm/1 -> MTQR_RrPosRateLimitDecE_Z_Nm/1
  MTQR_RrPosRateLimitDecE_Z_Nm/1 -> VTQR_RrPosRateLimitDecE_Nm/1  "VTQR_RrPosRateLimitDecE_Nm"

== system tqdtqr_rebuild_V3/Input_Convert/Main function/Front//Rear zero point transfer/Positive Rate limit Determination1/VTQR_RrPosRateLimitDecN_Nm ==
  VTQD_TqTargetShaftSpd_rpm : Inport
  VTQR_REDUWhlTqReqSmoothDelay_Nm : Inport  Port=2
  Action Port : ActionPort  ActionPortLabel=if(u1~= 0)
  MTQR_RrPosRateLimitDecN_Z_Nm : Lookup_n-D  BreakpointsForDimension1=ATQR_RrPosRateLimitIncN_Y_Nm  BreakpointsForDimension2=ATQR_RrPosRateLimitIncN_X_rpm  Table=MTQR_RrPosRateLimitDecN_Z_Nm  ExtrapMethod=Clip  UseLastTableValue=on  InternalRulePriority=Speed  RndMeth=Simplest  InputSameDT=on
      settings: InputPortMap=u0,u1
  VTQR_RrPosRateLimitDecN_Nm : Outport
  wires:
  VTQD_TqTargetShaftSpd_rpm/1 -> MTQR_RrPosRateLimitDecN_Z_Nm/2
  VTQR_REDUWhlTqReqSmoothDelay_Nm/1 -> MTQR_RrPosRateLimitDecN_Z_Nm/1
  MTQR_RrPosRateLimitDecN_Z_Nm/1 -> VTQR_RrPosRateLimitDecN_Nm/1  "VTQR_RrPosRateLimitDecN_Nm"

== system tqdtqr_rebuild_V3/Input_Convert/Main function/Front//Rear zero point transfer/Positive Rate limit Determination1/VTQR_RrPosRateLimitDecS_Nm ==
  VTQD_TqTargetShaftSpd_rpm : Inport
  VTQR_REDUWhlTqReqSmoothDelay_Nm : Inport  Port=2
  Action Port : ActionPort  ActionPortLabel=elseif( u3 ~= 0)
  MTQR_RrPosRateLimitDecE_Z_Nm : Lookup_n-D  BreakpointsForDimension1=ATQR_RrPosRateLimitIncN_Y_Nm  BreakpointsForDimension2=ATQR_RrPosRateLimitIncN_X_rpm  Table=MTQR_RrPosRateLimitDecS_Z_Nm  ExtrapMethod=Clip  UseLastTableValue=on  InternalRulePriority=Speed  RndMeth=Simplest  InputSameDT=on
      settings: InputPortMap=u0,u1
  VTQR_RrPosRateLimitDecS_Nm : Outport
  wires:
  VTQR_REDUWhlTqReqSmoothDelay_Nm/1 -> MTQR_RrPosRateLimitDecE_Z_Nm/1
  VTQD_TqTargetShaftSpd_rpm/1 -> MTQR_RrPosRateLimitDecE_Z_Nm/2
  MTQR_RrPosRateLimitDecE_Z_Nm/1 -> VTQR_RrPosRateLimitDecS_Nm/1  "VTQR_RrPosRateLimitDecS_Nm"

== system tqdtqr_rebuild_V3/Input_Convert/Main function/Front//Rear zero point transfer/Positive Rate limit Determination1/VTQR_RrPosRateLimitIncE_Nm ==
  VTQD_TqTargetShaftSpd_rpm : Inport
  VTQR_REDUWhlTqReqSmoothDelay_Nm : Inport  Port=2
  Action Port : ActionPort  ActionPortLabel=elseif(u2 ~= 0)
  MTQR_RrPosRateLimitIncE_Z_Nm : Lookup_n-D  BreakpointsForDimension1=ATQR_RrPosRateLimitIncN_Y_Nm  BreakpointsForDimension2=ATQR_RrPosRateLimitIncN_X_rpm  Table=MTQR_RrPosRateLimitIncE_Z_Nm  ExtrapMethod=Clip  UseLastTableValue=on  InternalRulePriority=Speed  RndMeth=Simplest  InputSameDT=on
      settings: InputPortMap=u0,u1
  VTQR_RrPosRateLimitIncE_Nm : Outport
  wires:
  VTQD_TqTargetShaftSpd_rpm/1 -> MTQR_RrPosRateLimitIncE_Z_Nm/2
  VTQR_REDUWhlTqReqSmoothDelay_Nm/1 -> MTQR_RrPosRateLimitIncE_Z_Nm/1
  MTQR_RrPosRateLimitIncE_Z_Nm/1 -> VTQR_RrPosRateLimitIncE_Nm/1  "VTQR_RrPosRateLimitIncE_Nm"

== system tqdtqr_rebuild_V3/Input_Convert/Main function/Front//Rear zero point transfer/Positive Rate limit Determination1/VTQR_RrPosRateLimitIncN_Nm ==
  VTQD_TqTargetShaftSpd_rpm : Inport
  VTQR_REDUWhlTqReqSmoothDelay_Nm : Inport  Port=2
  Action Port : ActionPort  ActionPortLabel=if(u1~= 0)
  MTQR_RrPosRateLimitIncN_Z_Nm : Lookup_n-D  BreakpointsForDimension1=ATQR_RrPosRateLimitIncN_Y_Nm  BreakpointsForDimension2=ATQR_RrPosRateLimitIncN_X_rpm  Table=MTQR_RrPosRateLimitIncN_Z_Nm  ExtrapMethod=Clip  UseLastTableValue=on  InternalRulePriority=Speed  RndMeth=Simplest  InputSameDT=on
      settings: InputPortMap=u0,u1
  VTQR_RrPosRateLimitIncN_Nm : Outport
  wires:
  VTQD_TqTargetShaftSpd_rpm/1 -> MTQR_RrPosRateLimitIncN_Z_Nm/2
  VTQR_REDUWhlTqReqSmoothDelay_Nm/1 -> MTQR_RrPosRateLimitIncN_Z_Nm/1
  MTQR_RrPosRateLimitIncN_Z_Nm/1 -> VTQR_RrPosRateLimitIncN_Nm/1  "VTQR_RrPosRateLimitIncN_Nm"

== system tqdtqr_rebuild_V3/Input_Convert/Main function/Front//Rear zero point transfer/Positive Rate limit Determination1/VTQR_RrPosRateLimitIncS_Nm ==
  VTQD_TqTargetShaftSpd_rpm : Inport
  VTQR_REDUWhlTqReqSmoothDelay_Nm : Inport  Port=2
  Action Port : ActionPort  ActionPortLabel=elseif( u3 ~= 0)
  MTQR_RrPosRateLimitIncS_Z_Nm : Lookup_n-D  BreakpointsForDimension1=ATQR_RrPosRateLimitIncN_Y_Nm  BreakpointsForDimension2=ATQR_RrPosRateLimitIncN_X_rpm  Table=MTQR_RrPosRateLimitIncS_Z_Nm  ExtrapMethod=Clip  UseLastTableValue=on  InternalRulePriority=Speed  RndMeth=Simplest  InputSameDT=on
      settings: InputPortMap=u0,u1
  VTQR_RrPosRateLimitIncS_Nm : Outport
  wires:
  VTQR_REDUWhlTqReqSmoothDelay_Nm/1 -> MTQR_RrPosRateLimitIncS_Z_Nm/1
  VTQD_TqTargetShaftSpd_rpm/1 -> MTQR_RrPosRateLimitIncS_Z_Nm/2
  MTQR_RrPosRateLimitIncS_Z_Nm/1 -> VTQR_RrPosRateLimitIncS_Nm/1  "VTQR_RrPosRateLimitIncS_Nm"

== system tqdtqr_rebuild_V3/Input_Convert/Signal function/Regen level define/Regen Level Switch Botton/RegenDOWN ==
  note: IF PRESS BOTH then nothing happen
  note: If press time more then Long press's limit then go Long press only. Else go short press only. Else if no press.
  note: Long press or Short press
  note: IF PRESS BOTH then nothing happen
  task_time_s : Inport
  SWC_RegenUp : Inport  Port=2
  SWC_RegenDOWN : Inport  Port=3
  AND : Logic  AllPortsSameDT=off  OutDataTypeStr=boolean
  AND1 : Logic  AllPortsSameDT=off  OutDataTypeStr=boolean
  AND2 : Logic  AllPortsSameDT=off  OutDataTypeStr=boolean
  Constant{1..2,4,7,10} (5 alike) : Constant  Value=FALSE
  Constant3 : Constant  Value=KTQD_RegShortPLim_s
  Default 3 sec : Constant  Value=KTQD_RegLongPLim_s
  DelayEnable_LONG_PRESS : hcu_lib/Basic_Blocks/DelayEnable
  DelayEnable_SHORT_PRESS : hcu_lib/Basic_Blocks/DelayEnable
  Detect Decrease1 : simulink/Logic and Bit Operations/Detect Decrease  vinit=boolean(0)  OutDataTypeStr=boolean
  Detect Decrease2 : simulink/Logic and Bit Operations/Detect Decrease  vinit=boolean(0)  OutDataTypeStr=boolean
  Detect Increase : simulink/Logic and Bit Operations/Detect Increase  vinit=boolean(0)  OutDataTypeStr=boolean
  NOT : Logic  Operator=NOT  AllPortsSameDT=off  OutDataTypeStr=boolean
  NOT1 : Logic  Operator=NOT  AllPortsSameDT=off  OutDataTypeStr=boolean
  SR_Latch : hcu_lib/Basic_Blocks/SR_Latch
  Switch{1..5} (5 alike) : Switch  Criteria=u2 ~= 0
      Switch2 settings: AttributesFormatString=%<Criteria>
      Switch3 settings: AttributesFormatString=%<Criteria>
      Switch4 settings: AttributesFormatString=%<Criteria>
      Switch5 settings: AttributesFormatString=%<Criteria>
  SWC_RegenDownShort_flg : Outport
  VTQD_RegenDownLongP_flg : Outport  Port=2
  wires:
  task_time_s/1 -> [task_time_s]
  Detect Increase/1 -> VTQD_RegenDownLongP_flg/1
  [task_time_s] -> DelayEnable_LONG_PRESS/3
  Default 3 sec/1 -> DelayEnable_LONG_PRESS/2
  [task_time_s] -> DelayEnable_SHORT_PRESS/3
  Constant3/1 -> DelayEnable_SHORT_PRESS/2
  DelayEnable_SHORT_PRESS/1 -> Detect Decrease2/1
  Constant7/1 -> Switch1/3
  DelayEnable_LONG_PRESS/1 -> Switch1/1, Switch1/2
  Switch1/1 -> Switch3/3
  [Short_press_falling_Edge] -> AND/1
  [Long_press] -> Detect Decrease1/1, Detect Increase/1
  Constant10/1 -> Switch2/1
  [Short_press_falling_Edge] -> Switch2/3
  Switch5/1 -> DelayEnable_SHORT_PRESS/1, DelayEnable_LONG_PRESS/1
  AND/1 -> Switch2/2
  Switch2/1 -> SWC_RegenDownShort_flg/1
  Switch3/1 -> [Long_press]
  SWC_RegenUp/1 -> [SWC_RegenUp]
  SWC_RegenDOWN/1 -> [SWC_RegenDOWN]
  [PRESS_BOTH] -> Switch3/2
  [SWC_RegenDOWN] -> AND1/2
  [SWC_RegenUp] -> AND1/1
  AND1/1 -> SR_Latch/1
  Constant1/1 -> Switch3/1
  Constant2/1 -> Switch4/1
  [PRESS_BOTH] -> Switch4/2
  Detect Decrease2/1 -> Switch4/3
  Switch4/1 -> [Short_press_falling_Edge]
  [SWC_RegenDOWN] -> Switch5/3
  [PRESS_BOTH] -> Switch5/2
  Constant4/1 -> Switch5/1
  [SWC_RegenUp] -> NOT/1
  [SWC_RegenDOWN] -> NOT1/1
  NOT/1 -> AND2/1
  NOT1/1 -> AND2/2
  AND2/1 -> SR_Latch/2
  SR_Latch/1 -> [PRESS_BOTH]
  Detect Decrease1/1 -> AND/2

== system tqdtqr_rebuild_V3/Input_Convert/Signal function/Regen level define/Regen Level Switch Botton/RegenUP ==
  note: IF PRESS BOTH then nothing happen
  note: If press time more then Long press's limit then go Long press only. Else go short press only. Else if no press.
  note: Long press or Short press
  note: IF PRESS BOTH then nothing happen
  task_time_s : Inport
  SWC_RegenUp : Inport  Port=2
  SWC_RegenDOWN : Inport  Port=3
  AND : Logic  AllPortsSameDT=off  OutDataTypeStr=boolean
  AND1 : Logic  AllPortsSameDT=off  OutDataTypeStr=boolean
  AND2 : Logic  AllPortsSameDT=off  OutDataTypeStr=boolean
  Constant{1..2,4,7,10} (5 alike) : Constant  Value=FALSE
  Constant3 : Constant  Value=KTQD_RegShortPLim_s
  Default 3 sec : Constant  Value=KTQD_RegLongPLim_s
  DelayEnable_LONG_PRESS : hcu_lib/Basic_Blocks/DelayEnable
  DelayEnable_SHORT_PRESS : hcu_lib/Basic_Blocks/DelayEnable
  Detect Decrease1 : simulink/Logic and Bit Operations/Detect Decrease  vinit=boolean(0)  OutDataTypeStr=boolean
  Detect Decrease2 : simulink/Logic and Bit Operations/Detect Decrease  vinit=boolean(0)  OutDataTypeStr=boolean
  Detect Increase : simulink/Logic and Bit Operations/Detect Increase  vinit=boolean(0)  OutDataTypeStr=boolean
  NOT : Logic  Operator=NOT  AllPortsSameDT=off  OutDataTypeStr=boolean
  NOT1 : Logic  Operator=NOT  AllPortsSameDT=off  OutDataTypeStr=boolean
  SR_Latch : hcu_lib/Basic_Blocks/SR_Latch
  Switch{1..5} (5 alike) : Switch  Criteria=u2 ~= 0
      settings: AttributesFormatString=%<Criteria>
  SWC_RegenUpShort_flg : Outport
  VTQD_RegenUpLongP_flg : Outport  Port=2
  wires:
  task_time_s/1 -> [task_time_s]
  Detect Increase/1 -> VTQD_RegenUpLongP_flg/1
  [task_time_s] -> DelayEnable_LONG_PRESS/3
  Default 3 sec/1 -> DelayEnable_LONG_PRESS/2
  [task_time_s] -> DelayEnable_SHORT_PRESS/3
  Constant3/1 -> DelayEnable_SHORT_PRESS/2
  DelayEnable_SHORT_PRESS/1 -> Detect Decrease2/1
  Constant7/1 -> Switch1/3
  DelayEnable_LONG_PRESS/1 -> Switch1/1, Switch1/2
  Switch1/1 -> Switch3/3
  [Short_press_falling_Edge] -> AND/1
  [Long_press] -> Detect Decrease1/1, Detect Increase/1
  Constant10/1 -> Switch2/1
  [Short_press_falling_Edge] -> Switch2/3
  Switch5/1 -> DelayEnable_SHORT_PRESS/1, DelayEnable_LONG_PRESS/1
  AND/1 -> Switch2/2
  Switch2/1 -> SWC_RegenUpShort_flg/1
  Switch3/1 -> [Long_press]
  SWC_RegenUp/1 -> [SWC_RegenUp]
  SWC_RegenDOWN/1 -> [SWC_RegenDOWN]
  [PRESS_BOTH] -> Switch3/2
  [SWC_RegenDOWN] -> AND1/2
  [SWC_RegenUp] -> AND1/1
  AND1/1 -> SR_Latch/1
  Constant1/1 -> Switch3/1
  Constant2/1 -> Switch4/1
  [PRESS_BOTH] -> Switch4/2
  Detect Decrease2/1 -> Switch4/3
  Switch4/1 -> [Short_press_falling_Edge]
  [SWC_RegenUp] -> Switch5/3
  [PRESS_BOTH] -> Switch5/2
  Constant4/1 -> Switch5/1
  [SWC_RegenUp] -> NOT/1
  [SWC_RegenDOWN] -> NOT1/1
  NOT/1 -> AND2/1
  NOT1/1 -> AND2/2
  AND2/1 -> SR_Latch/2
  SR_Latch/1 -> [PRESS_BOTH]
  Detect Decrease1/1 -> AND/2

== system tqdtqr_rebuild_V3/Input_Convert/Signal function/SWC1 SWC2 status/SWC2_Subsystem/L_ScrollPress Behavior ==
  note: Long press or Short press
  note: If press time more then Long press's limit then go Long press only. Else go short press only. Else if no press.
  VTQD_SWC2LScrollPressSta_flg : Inport
  TASK_TIME : Inport  Port=2
  VVMC_MSACtrlSta_enum : Inport  Port=3
  AND : Logic  AllPortsSameDT=off  OutDataTypeStr=boolean
  Constant10 : Constant  Value=FALSE
  Constant3 : Constant  Value=KTQD_SpdModeShortPLim_s
  Constant7 : Constant  Value=FALSE
  Default 3 sec : Constant  Value=KTQD_SpdModeLongPLim_s
  Default 3 sec1 : Constant  Value=KTQD_SpdModeLongPCancelLim_s
  Default 3 sec2 : Constant  Value=ENUM_ADASMSASTA_ACTIVE
  Default 3 sec3 : Constant  Value=ENUM_ADASMSASTA_UNLIMIT
  DelayEnable_LONG_PRESS : hcu_lib/Basic_Blocks/DelayEnable
  DelayEnable_SHORT_PRESS : hcu_lib/Basic_Blocks/DelayEnable
  Detect Decrease1 : simulink/Logic and Bit Operations/Detect Decrease  vinit=boolean(0)  OutDataTypeStr=boolean
  Detect Decrease2 : simulink/Logic and Bit Operations/Detect Decrease  vinit=0.0  OutDataTypeStr=boolean
  Detect Increase : simulink/Logic and Bit Operations/Detect Increase  vinit=boolean(0)  OutDataTypeStr=boolean
  OR : Logic  Operator=OR  AllPortsSameDT=off  OutDataTypeStr=boolean
  Relational Operator : RelationalOperator  Operator===  OutDataTypeStr=boolean  RndMeth=Simplest
  Relational Operator1 : RelationalOperator  Operator===  OutDataTypeStr=boolean  RndMeth=Simplest
  Switch : Switch  Criteria=u2 ~= 0
      settings: AttributesFormatString=%<Criteria>
  Switch1 : Switch  Criteria=u2 ~= 0
      settings: AttributesFormatString=%<Criteria>
  Switch2 : Switch  Criteria=u2 ~= 0
      settings: AttributesFormatString=%<Criteria>
  VTQD_LScrollPressShort_flg : Outport
  "VTQD_LScrollPressLong_flg\t" : Outport  Port=2
  wires:
  Default 3 sec1/1 -> Switch/1
  Default 3 sec/1 -> Switch/3
  OR/1 -> Switch/2
  Relational Operator1/1 -> OR/2
  Relational Operator/1 -> OR/1
  Default 3 sec3/1 -> Relational Operator1/2
  VVMC_MSACtrlSta_enum/1 -> Relational Operator/1, Relational Operator1/1
  Default 3 sec2/1 -> Relational Operator/2
  TASK_TIME/1 -> [TASK_TIME]
  Switch1/1 -> [Long_press]
  Detect Decrease2/1 -> [Short_press_falling_Edge]
  Detect Decrease1/1 -> AND/2
  VTQD_SWC2LScrollPressSta_flg/1 -> [VTQD_SWC2LScrollPressSta_flg]
  Switch2/1 -> VTQD_LScrollPressShort_flg/1
  AND/1 -> Switch2/2
  [VTQD_SWC2LScrollPressSta_flg] -> DelayEnable_LONG_PRESS/1, DelayEnable_SHORT_PRESS/1
  [Short_press_falling_Edge] -> Switch2/3
  Constant10/1 -> Switch2/1
  [Long_press] -> Detect Increase/1, Detect Decrease1/1
  [Short_press_falling_Edge] -> AND/1
  DelayEnable_LONG_PRESS/1 -> Switch1/2, Switch1/1
  Constant7/1 -> Switch1/3
  DelayEnable_SHORT_PRESS/1 -> Detect Decrease2/1
  Constant3/1 -> DelayEnable_SHORT_PRESS/2
  [TASK_TIME] -> DelayEnable_SHORT_PRESS/3
  Switch/1 -> DelayEnable_LONG_PRESS/2
  [TASK_TIME] -> DelayEnable_LONG_PRESS/3
  Detect Increase/1 -> "VTQD_LScrollPressLong_flg\t"/1
